simulink model "SCARA"  (R2018a)
settings: Solver=VariableStepAuto  StartTime=0.0  StopTime=10.0  RelTol=1e-3
model workspace: external: MATLAB File C:\Users\1511 MXTI\Desktop\CEFET\ROBÓTICA\SCARA 4\SCARA4_DataFile1.m (data not in the file)
undefined symbols (not defined in the file or in its folder): smiData, X, Y, Z
libraries: sm_lib x20, nesl_utility x9
(part 1 of 2)
settings Model: Creator=1511 MXTI  LastModifiedBy=1511 MXTI

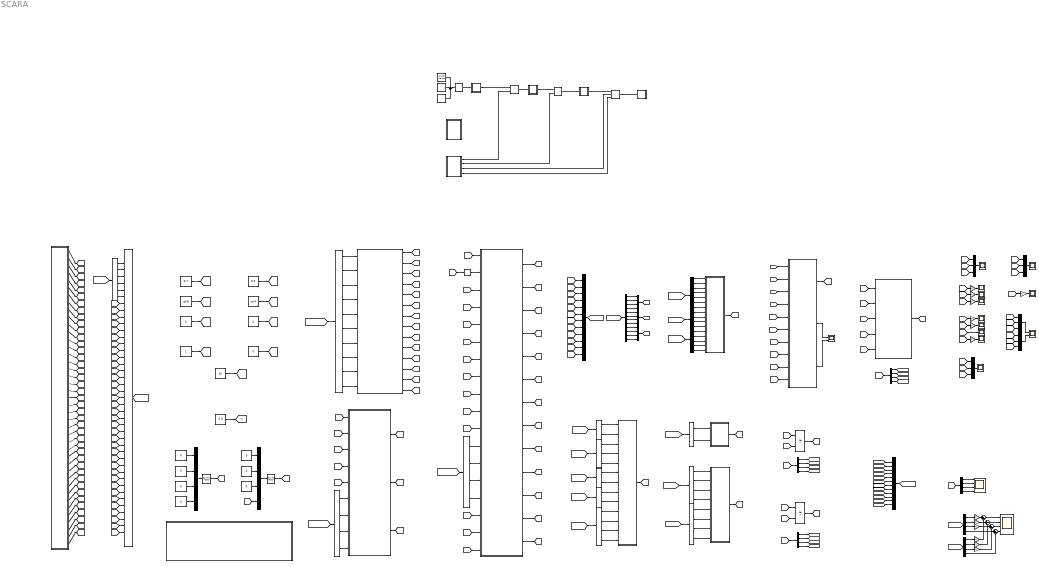
== system SCARA ==
  note: Disciplina: Robótica (GELE0931) 2020_2 T.A
      |
      | Professor: Luciano Raptopoulos
      | luciano.raptopoulos@cefet-rj.br
      |
      | Alunos:
      | Felipe Leite da Fonseca
      | Luan Almeida de Oliveira
      |
      | felipe.leite@aluno.cefet-rj.br
      |
      | luan.almeida@aluno.cefet-rj.br
  note: VELOCIDADES INICIAIS DAS JUNTAS
  note: TORQUE NAS JUNTAS
  note: DADOS DO MODELO
  note: TEST POSIÇÃO DA FERRAMENTA
  note: ANGULO DA FERRAMENTA
  note: Qs DESEJADOS
  note: POSIÇAO DA FERRAMENTA
  note: ACELERAÇÕES DA FERRAMENTA
  note: VELOCIDADES DA FERRAMENTA
  note: ANGULO DA FERRAMENTA
  note: DADOS DE ENTRADA DA TAREFA
  note: POSIÇÕES INICIAIS DAS JUNTAS
  note: VELOCIDADES SIMULADAS DAS JUNTAS
  note: POSIÇÕES SIMULADAS DAS JUNTAS
  note: CÁLCULO DA TRAJETÓRIA
  note: CINEMÁTICA INVERSA
  note: q dq ddq DESEJADOS
  note: q dq ddq SIMULADOS
  note: MODELO 3D DO SCARA
  note: SCARA COMPLETO
  note: TEMPO DE ASSENTAMENTO
  note: ERRO DAS JUNTAS
  note: PLOTAGENS
  note: PARAMETROS INICIAIS
  note: PARAMETROS FINAIS
  note: ALTURA DA FERRAMENTA EM RELAÇÃO AO SOLO
  note: DESEJADO
  note: SIMULADO
  note: INSTRUÇÕES DE UTILIZAÇÃO:
      |
      | Todos os grandes blocos utilizados para projetar o controle do robô SCARA apresentado foram separados nas áreas abaixo devidamente intituladas.
      |
      | As entradas estão dispostas na área em AZUL nos blocos de constante em VERDE .
      |
      | As saídas préviamente requisitadas serão abertas automáticamente ao rodar a simulação, como os torques, força e erros das juntas.
      |
      | Outras plotagens previamente definidas se encontram na área em AMARELO .
  note: M
  note: CONTROLADOR
  note: TESTE DA CINEMÁTICA
  note: TRATAMENTO DAS ENTRADAS
  note: DADOS DE ENTRADA DO CONTROLADOR
  note: PLANTA
  note: INTEGRAÇÕES
  note: G & D
  note: H
  Alpha final (rad) : Constant  Value=0
  Alpha inicial (rad) : Constant  Value=0
  Altura final (m) : Constant  Value=0
  Altura inicial (m) : Constant
  BASE_SCARA_2_RIGID : Subsystem
  Bus Creator : BusCreator  Inputs=12
  Bus Creator4 : BusCreator  Inputs=12
  Bus Creator5 : BusCreator  Inputs=41
  Bus Creator6 : BusCreator  Inputs=4
  Bus Creator7 : BusCreator  Inputs=4
  Bus Selector : BusSelector  OutputSignals=t,tf,R0,Rf,teta0,tetaf,alfa0,alfaf,h0,hf
  Bus Selector1 : BusSelector  OutputSignals=q1,q2,q4,q3
  Bus Selector10 : BusSelector  OutputSignals=L0,L1,e1,L2,e2,L3
  Bus Selector11 : BusSelector  OutputSignals=xG1,xG2,xG3,yG1,yG2,yG3
  Bus Selector12 : BusSelector  OutputSignals=signal2,signal4
  Bus Selector13 : BusSelector  OutputSignals=L1,L2
  Bus Selector14 : BusSelector  OutputSignals=signal1,signal2,signal4
  Bus Selector15 : BusSelector  OutputSignals=m2,m3
  Bus Selector16 : BusSelector  OutputSignals=xG2,xG3,yG2,yG3
  Bus Selector17 : BusSelector  OutputSignals=g,m3
  Bus Selector18 : BusSelector  OutputSignals=c1,c2,c3,c4
  Bus Selector19 : BusSelector  OutputSignals=signal2,signal4
  Bus Selector2 : BusSelector  OutputSignals=L0,L1,L2,e1
  Bus Selector20 : BusSelector  OutputSignals=signal5,signal6,signal7,signal8
  Bus Selector21 : BusSelector  OutputSignals=q1,q2,q3,q4,dq1d,dq2d,dq3d,dq4d,d2q1d,d2q2d,d2q3d,d2q4d
  Bus Selector3 : BusSelector  OutputSignals=signal1,signal2,signal4,signal3
  Bus Selector5 : BusSelector  OutputSignals=L0,L1,e1,L2
  Bus Selector9 : BusSelector  OutputSignals=Izz1,Izz2,Izz3,L1,L2,m1,m2,m3
  Bus to Vector1 : BusToVector
  Bus to Vector2 : BusToVector
  Cylindrical : sm_lib/Joints/Cylindrical Joint  SenseConstraintForce=off  SenseConstraintForceX=off  SenseConstraintForceY=off  SenseConstraintForceZ=off  SenseConstraintTorque=off  SenseConstraintTorqueX=off  SenseConstraintTorqueY=off  SenseConstraintTorqueZ=off  SenseTotalForce=off  SenseTotalForceX=off  SenseTotalForceY=off  SenseTotalForceZ=off  SenseTotalTorque=off  SenseTotalTorqueX=off  SenseTotalTorqueY=off  SenseTotalTorqueZ=off  CompositeWrenchDir=FollowerOnBase  CompositeWrenchFrame=BaseFrame  PzEquilibriumPosition=0  PzEquilibriumPositionUnits=m  PzSpringStiffness=0  PzSpringStiffnessUnits=N/m  PzDampingCoefficient=0  PzDampingCoefficientUnits=N/(m/s)  PzTorqueActuationMode=ComputedTorque  PzMotionActuationMode=InputMotion  PzSensePosition=off  PzSenseVelocity=off  PzSenseAcceleration=off  PzSenseTorqueForce=off  PzPositionTargetSpecify=on  PzPositionTargetPriority=Low  PzPositionTargetValue=smiData.CylindricalJoint(1).Pz.Pos  PzPositionTargetValueUnits=mm  PzVelocityTargetSpecify=off  PzVelocityTargetPriority=High  PzVelocityTargetValue=0  PzVelocityTargetValueUnits=m/s  RzEquilibriumPosition=0  RzEquilibriumPositionUnits=rad  RzSpringStiffness=0  RzSpringStiffnessUnits=N*m/rad  RzDampingCoefficient=0  RzDampingCoefficientUnits=N*m/(rad/s)  RzTorqueActuationMode=ComputedTorque  RzMotionActuationMode=InputMotion  RzSensePosition=off  RzSenseVelocity=off  RzSenseAcceleration=off  RzSenseTorqueForce=off  RzPositionTargetSpecify=on  RzPositionTargetPriority=Low  RzPositionTargetValue=smiData.CylindricalJoint(1).Rz.Pos  RzPositionTargetValueUnits=deg  RzVelocityTargetSpecify=off  RzVelocityTargetPriority=High  RzVelocityTargetValue=0  RzVelocityTargetValueUnits=deg/s
  D : MATLAB Function  TreatAsAtomicUnit=on
  DQ1S0 : Constant  Value=0
  DQ2S0 : Constant  Value=0
  DQ3S0 : Constant  Value=0
  DQ4S0 : Constant  Value=0
  Demux{,3..5} (4 alike) : Demux
  Duração da tarefa (s) : Constant  Value=10
  ELO_01_SCARA_1_RIGID : Subsystem
  ELO_02_SCARA_1_RIGID : Subsystem
  ELO_03_SCARA_1_RIGID : Subsystem
  G : MATLAB Function  TreatAsAtomicUnit=on
  Gain{,1..10,14..15} (13 alike) : Gain  Gain=180/pi
  H : MATLAB Function  TreatAsAtomicUnit=on
  Integrator2 : Integrator  InitialConditionSource=external  InitialCondition=[0 0 0 0]
  Integrator3 : Integrator  InitialConditionSource=external  InitialCondition=[0 0 0 0]
  JUNTAS DESEJADAS : Subsystem
  JUNTAS SIMULADAS : Subsystem
  M : MATLAB Function  TreatAsAtomicUnit=on
  MATLAB Function1 : MATLAB Function  TreatAsAtomicUnit=on
  MATLAB Function4 : MATLAB Function  TreatAsAtomicUnit=on
  MATLAB Function5 : MATLAB Function  TreatAsAtomicUnit=on
  MATLAB Function6 : MATLAB Function  TreatAsAtomicUnit=on
  MATLAB Function7 : MATLAB Function  TreatAsAtomicUnit=on
  MechanismConfiguration : sm_lib/Utilities/Mechanism Configuration  UniformGravity=Constant  GravityVector=[0 -9.80665 0]  GravityUnits=m/s^2  LinearizationDelta=0.001
  Memory : Memory
  Mux{,1..2,4..5} (5 alike) : Mux  Inputs=3
  Mux3 : Mux
  Mux7 : Mux
  Mux8 : Mux
  Q1S0 : Constant  Value=0
  Q2S0 : Constant  Value=0
  Q3S0 : Constant  Value=0
  Raio final (m) : Constant  Value=0.5
  Raio inicial (m) : Constant  Value=0.7
  Revolute : sm_lib/Joints/Revolute Joint  SenseConstraintForce=off  SenseConstraintForceX=off  SenseConstraintForceY=off  SenseConstraintForceZ=off  SenseConstraintTorque=off  SenseConstraintTorqueX=off  SenseConstraintTorqueY=off  SenseConstraintTorqueZ=off  SenseTotalForce=off  SenseTotalForceX=off  SenseTotalForceY=off  SenseTotalForceZ=off  SenseTotalTorque=off  SenseTotalTorqueX=off  SenseTotalTorqueY=off  SenseTotalTorqueZ=off  CompositeWrenchDir=FollowerOnBase  CompositeWrenchFrame=BaseFrame  EquilibriumPosition=0  EquilibriumPositionUnits=rad  SpringStiffness=0  SpringStiffnessUnits=N*m/rad  DampingCoefficient=0  DampingCoefficientUnits=N*m/(rad/s)  TorqueActuationMode=ComputedTorque  MotionActuationMode=InputMotion  SensePosition=off  SenseVelocity=off  SenseAcceleration=off  SenseTorqueForce=off  PositionTargetSpecify=on  PositionTargetPriority=Low  PositionTargetValue=smiData.RevoluteJoint(1).Rz.Pos  PositionTargetValueUnits=deg  VelocityTargetSpecify=off  VelocityTargetPriority=High  VelocityTargetValue=0  VelocityTargetValueUnits=deg/s
  Revolute1 : sm_lib/Joints/Revolute Joint  SenseConstraintForce=off  SenseConstraintForceX=off  SenseConstraintForceY=off  SenseConstraintForceZ=off  SenseConstraintTorque=off  SenseConstraintTorqueX=off  SenseConstraintTorqueY=off  SenseConstraintTorqueZ=off  SenseTotalForce=off  SenseTotalForceX=off  SenseTotalForceY=off  SenseTotalForceZ=off  SenseTotalTorque=off  SenseTotalTorqueX=off  SenseTotalTorqueY=off  SenseTotalTorqueZ=off  CompositeWrenchDir=FollowerOnBase  CompositeWrenchFrame=BaseFrame  EquilibriumPosition=0  EquilibriumPositionUnits=rad  SpringStiffness=0  SpringStiffnessUnits=N*m/rad  DampingCoefficient=0  DampingCoefficientUnits=N*m/(rad/s)  TorqueActuationMode=ComputedTorque  MotionActuationMode=InputMotion  SensePosition=off  SenseVelocity=off  SenseAcceleration=off  SenseTorqueForce=off  PositionTargetSpecify=on  PositionTargetPriority=Low  PositionTargetValue=smiData.RevoluteJoint(2).Rz.Pos  PositionTargetValueUnits=deg  VelocityTargetSpecify=off  VelocityTargetPriority=High  VelocityTargetValue=0  VelocityTargetValueUnits=deg/s
  Scope{,1..6,8..9,18..19} (11 alike) : Scope
  Scope10 : Scope  NumInputPorts=2
  Scope11 : Scope  NumInputPorts=4
  Scope15 : Scope  NumInputPorts=4
  Scope7 : Scope  NumInputPorts=2
  Solver Configuration : nesl_utility/Solver Configuration  PhysicalDomain=network_engine_domain  SubClassName=solver  LeftPortType=input  RightPortType=generic  Tones=[]  Harmonics=[]  SimulateNoise=off  Profile=off  UseLocalSampling=off  EnableSwitchedLinearOptims=on  FrequencyDomain=off  UseCCode=off  RelTol=0.001  AbsTol=1e-06  MinStep=1e-09  ToWorkspace=off  RevertToSquareIcSolve=off  NumHomotopyIterations=100  PhasorMode=off  PhasorModeNumHarmonics=1  DoDC=off  ResidualTolerance=1e-09  UseLocalSolver=off  LocalSolverChoice=NE_BACKWARD_EULER_ADVANCER  LocalSolverSampleTime=0.001  DoFixedCost=off  MaxNonlinIter=3  MaxModeIter=2  LinearAlgebra=Sparse  EquationFormulation=NE_TIME_EF  DelaysMemoryBudget=1024  AutomaticFiltering=on  FilteringTimeConstant=0.001
  Sum{,1..3} (4 alike) : Sum  Inputs=|+-
  TEMPO DE ASSENTAMENTO(s) : Constant  Value=0.5
  TRAMENTO DAS ENTRADAS : Subsystem
  Theta final (rad) : Constant  Value=-pi/4  OutMin=[-2*pi]  OutMax=[2*pi]
  Theta inicial (rad) : Constant  Value=-pi/8  OutMin=[-2*pi]  OutMax=[2*pi]
  Transform : sm_lib/Frames and Transforms/Rigid Transform  TranslationMethod=Cartesian  TranslationStandardOffset=0  TranslationLengthUnit=mm  TranslationStandardAxis=+Z  TranslationCartesianOffset=smiData.RigidTransform(7).translation  TranslationROffset=0  TranslationROffsetUnits=m  TranslationZOffset=0  TranslationZOffsetUnits=m  TranslationThetaOffset=0  TranslationThetaOffsetUnits=deg  RotationMethod=ArbitraryAxis  RotationAngleUnits=rad  RotationStandardAxis=+Z  RotationAngle=smiData.RigidTransform(7).angle  RotationArbitraryAxis=smiData.RigidTransform(7).axis  FollAlignAxisA=+X  BaseAlignAxisA=+Y  FollAlignAxisB=+Y  BaseAlignAxisB=+Z  RotationSequenceAxes=FollowerAxes  RotationSequence=XYX  RotationSequenceAngles=[0 0 0]  RotationSequenceAnglesUnits=deg  RotationMatrix=[1 0 0; 0 1 0; 0 0 1]
  VALORES : MATLAB Function  TreatAsAtomicUnit=on
  World : sm_lib/Frames and Transforms/World Frame
  tag scope: ALPHA_FINAL=global, ALPHA_INICIAL=global, ALTURA_FINAL=global, ALTURA_INICIAL=global, DURACAO_DA_TAREFA=global, L1i=global, L2i=global, L3i=global, LOi=global, P0s=global, RAIO_FINAL=global, RAIO_INICIAL=global, THETA_FINAL=global, THETA_INICIAL=global, Ts=global, V0s=global, c1=global, d2q1d=global, d2q2d=global, d2q3d=global, d2q4d=global, d2qs=global, ddy=global, dq1d=global, dq2d=global, dq3d=global, dq4d=global, dqs=global, e1i=global, e2i=global, horario=global, q1d=global, q2d=global, q3d=global, q4d=global, qd_dqd_d2qd=global, qs=global, qs_dqs_d2qs=global, t_x=global, t_y=global, t_z=global, teta=global, x=global, y=global, z=global
  wires:
  Bus Selector/5 -> MATLAB Function6/5(teta0)  "<teta0>"
  Bus Selector/8 -> MATLAB Function6/8(alfaf)  "<alfaf>"
  [INPUT] -> Bus Selector/1
  [x] -> MATLAB Function7/3(x)
  Bus Selector/1 -> MATLAB Function6/1(t)  "<t>"
  Bus Selector/6 -> MATLAB Function6/6(tetaf)  "<tetaf>"
  Bus Selector/3 -> MATLAB Function6/3(R0)  "<R0>"
  MATLAB Function6/5(z) -> [z]
  MATLAB Function6/13(dalfa) -> [dalfa]
  MATLAB Function6/1(horario) -> [horario]
  Bus Selector/2 -> MATLAB Function6/2(tf)  "<tf>"
  Bus Selector/4 -> MATLAB Function6/4(Rf)  "<Rf>"
  Bus Selector/7 -> MATLAB Function6/7(alfa0)  "<alfa0>"
  MATLAB Function6/11(ddz) -> [ddz]
  MATLAB Function6/6(dx) -> [dx]
  Bus Selector2/4 -> MATLAB Function7/15(e1)  "<e1>"
  MATLAB Function6/3(x) -> [x]
  MATLAB Function6/7(dy) -> [dy]
  MATLAB Function6/4(y) -> [y]
  MATLAB Function6/8(dz) -> [dz]
  [y] -> MATLAB Function7/4(y)
  MATLAB Function6/14(d2alfa) -> [ddalfa]
  Bus Selector2/2 -> MATLAB Function7/13(L1)  "<L1>"
  [alfa] -> MATLAB Function7/16(alfa)
  MATLAB Function6/2(teta) -> [teta]
  MATLAB Function6/9(ddx) -> [ddx]
  Bus Selector2/3 -> MATLAB Function7/14(L2)  "<L2>"
  [z] -> MATLAB Function7/5(z)
  MATLAB Function6/10(ddy) -> [ddy]
  MATLAB Function6/12(alfa) -> [alfa]
  Bus Selector2/1 -> MATLAB Function7/12(L0)  "<L0>"
  Memory/1 -> MATLAB Function7/2(phiAnterior)
  [phi] -> Memory/1
  [t_z] -> Mux5/3
  [t_x] -> Mux5/1
  [q2d] -> Gain4/1
  [t_y] -> Mux5/2
  [q4d] -> Gain2/1
  [z] -> Mux2/3
  Gain15/1 -> Scope4/1
  [y] -> Mux2/2
  Gain/1 -> Scope9/1
  Gain14/1 -> Scope3/1
  Gain1/1 -> Scope18/1
  Mux/1 -> Scope/1
  [ddz] -> Mux4/3
  Mux4/1 -> Scope2/1
  Gain2/1 -> Scope6/1
  [ddy] -> Mux4/2
  [ddx] -> Mux4/1
  [y] -> Mux/2
  Gain3/1 -> Scope19/1
  [x] -> Mux/1
  [dalfa] -> Gain1/1
  [dz] -> Mux1/3
  [dy] -> Mux1/2
  [q1d] -> Gain15/1
  Mux2/1 -> Scope7/1
  [dx] -> Mux1/1
  Mux1/1 -> Scope1/1
  [alfa] -> Gain/1
  Mux5/1 -> Scope7/2
  [z] -> Mux/3
  [x] -> Mux2/1
  [teta] -> Gain14/1
  [ddalfa] -> Gain3/1
  [q3d] -> Scope5/1
  Gain4/1 -> Scope8/1
  [q4d] -> MATLAB Function1/5(q4)
  Bus Selector5/1 -> MATLAB Function1/6(L0)  "<L0>"
  Bus Selector5/3 -> MATLAB Function1/8(e1)  "<e1>"
  [q3d] -> MATLAB Function1/4(q3)
  [q2d] -> MATLAB Function1/3(q2)
  Bus Selector5/2 -> MATLAB Function1/7(L1)  "<L1>"
  [DIMENSIONAL] -> Bus Selector5/1
  [horario] -> MATLAB Function1/1(horario)
  MATLAB Function1/1(x) -> [t_x]
  [q1d] -> MATLAB Function1/2(q1)
  MATLAB Function1/3(z) -> [t_z]
  Bus Selector5/4 -> MATLAB Function1/9(L2)  "<L2>"
  MATLAB Function1/2(y) -> [t_y]
  [q1d] -> Bus Creator4/1
  [q2d] -> Bus Creator4/2
  [q3d] -> Bus Creator4/3
  [q4d] -> Bus Creator4/4
  [dq1d] -> Bus Creator4/5
  [dq2d] -> Bus Creator4/6
  [dq3d] -> Bus Creator4/7
  [dq4d] -> Bus Creator4/8
  [d2q1d] -> Bus Creator4/9
  [d2q2d] -> Bus Creator4/10
  [d2q3d] -> Bus Creator4/11
  [d2q4d] -> Bus Creator4/12
  Bus Creator4/1 -> [qd_dqd_d2qd]
  Bus Selector14/2 -> H/4(dq2)  "<signal2>"
  Demux5/1 -> [d2q1s]
  Demux4/4 -> [q4s]
  Demux5/3 -> [d2q3s]
  [qs] -> MATLAB Function4/5(qs)
  Demux5/4 -> [d2q4s]
  Demux3/1 -> [dq1s]
  Demux5/2 -> [d2q2s]
  [dqs] -> MATLAB Function4/6(dqs)
  Demux3/3 -> [dq3s]
  Bus Selector14/1 -> H/3(dq1)  "<signal1>"
  Demux4/2 -> [q2s]
  Demux3/2 -> [dq2s]
  Demux4/3 -> [q3s]
  Demux4/1 -> [q1s]
  VALORES/2(L1i) -> [L1i]
  VALORES/3(e1i) -> [e1i]
  VALORES/4(L2i) -> [L2i]
  VALORES/5(e2i) -> [e2i]
  VALORES/6(L3i) -> [L3i]
  VALORES/7(c1) -> [c1]
  VALORES/8(c2) -> [c2]
  VALORES/9(c3) -> [c3]
  VALORES/10(c4) -> [c4]
  VALORES/11(g) -> [g]
  VALORES/12(m1) -> [m1]
  VALORES/13(xG1) -> [xG1]
  VALORES/14(yG1) -> [yG1]
  VALORES/15(zG1) -> [zG1]
  VALORES/16(Ixx1) -> [Ixx1]
  VALORES/17(Ixy1) -> [Ixy1]
  VALORES/18(Ixz1) -> [Ixz1]
  VALORES/19(Iyy1) -> [Iyy1]
  VALORES/20(Iyz1) -> [Iyz1]
  VALORES/21(Izz1) -> [Izz1]
  VALORES/22(m2) -> [m2]
  VALORES/23(xG2) -> [xG2]
  VALORES/24(yG2) -> [yG2]
  VALORES/25(zG2) -> [zG2]
  VALORES/26(Ixx2) -> [Ixx2]
  VALORES/27(Ixy2) -> [Ixy2]
  VALORES/28(Ixz2) -> [Ixz2]
  VALORES/29(Iyy2) -> [Iyy2]
  VALORES/30(Iyz2) -> [Iyz2]
  VALORES/31(Izz2) -> [Izz2]
  VALORES/32(m3) -> [m3]
  VALORES/41(Izz3) -> [Izz3]
  VALORES/40(Iyz3) -> [Iyz3]
  VALORES/39(Iyy3) -> [Iyy3]
  VALORES/38(Ixz3) -> [Ixz3]
  VALORES/37(Ixy3) -> [Ixy3]
  VALORES/36(Ixx3) -> [Ixx3]
  VALORES/35(zG3) -> [zG3]
  VALORES/34(yG3) -> [yG3]
  VALORES/33(xG3) -> [xG3]
  VALORES/1(LOi) -> [LOi]
  [c1] -> Bus Creator5/7
  [c2] -> Bus Creator5/8
  [c3] -> Bus Creator5/9
  [c4] -> Bus Creator5/10
  [g] -> Bus Creator5/11
  [m1] -> Bus Creator5/12
  [xG1] -> Bus Creator5/13
  [Ixz1] -> Bus Creator5/18
  [Ixy1] -> Bus Creator5/17
  [Ixx1] -> Bus Creator5/16
  [zG1] -> Bus Creator5/15
  [yG1] -> Bus Creator5/14
  [Iyy1] -> Bus Creator5/19
  [Iyz1] -> Bus Creator5/20
  [Izz1] -> Bus Creator5/21
  [m2] -> Bus Creator5/22
  [xG2] -> Bus Creator5/23
  [yG2] -> Bus Creator5/24
  [Ixx2] -> Bus Creator5/26
  [zG2] -> Bus Creator5/25
  [Ixy2] -> Bus Creator5/27
  [Ixz2] -> Bus Creator5/28
  [Iyy2] -> Bus Creator5/29
  [Iyz2] -> Bus Creator5/30
  [Izz2] -> Bus Creator5/31
  [m3] -> Bus Creator5/32
  [xG3] -> Bus Creator5/33
  [yG3] -> Bus Creator5/34
  [zG3] -> Bus Creator5/35
  [Ixx3] -> Bus Creator5/36
  [Ixy3] -> Bus Creator5/37
  [Ixz3] -> Bus Creator5/38
  [Iyy3] -> Bus Creator5/39
  [Iyz3] -> Bus Creator5/40
  [Izz3] -> Bus Creator5/41
  Bus Creator5/1 -> [ALL_IN]
  [ALL_IN] -> Bus Selector9/1
  [DIMENSIONAL] -> Bus Selector10/1
  Bus Selector10/1 -> Bus Creator5/1  "<L0>"
  Bus Selector10/2 -> Bus Creator5/2  "<L1>"
  Bus Selector10/3 -> Bus Creator5/3  "<e1>"
  Bus Selector10/4 -> Bus Creator5/4  "<L2>"
  Bus Selector10/5 -> Bus Creator5/5  "<e2>"
  Bus Selector10/6 -> Bus Creator5/6  "<L3>"
  Bus Selector9/1 -> M/1(Izz1)  "<Izz1>"
  Bus Selector9/2 -> M/2(Izz2)  "<Izz2>"
  Bus Selector9/3 -> M/3(Izz3)  "<Izz3>"
  Bus Selector9/4 -> M/4(L1)  "<L1>"
  Bus Selector9/5 -> M/5(L2)  "<L2>"
  Bus Selector9/6 -> M/6(m1)  "<m1>"
  Bus Selector9/7 -> M/7(m2)  "<m2>"
  Bus Selector9/8 -> M/8(m3)  "<m3>"
  [ALL_IN] -> Bus Selector11/1
  Bus Selector11/1 -> M/11(xG1)  "<xG1>"
  Bus Selector11/2 -> M/12(xG2)  "<xG2>"
  Bus Selector11/3 -> M/13(xG3)  "<xG3>"
  Bus Selector11/4 -> M/14(yG1)  "<yG1>"
  Bus Selector11/5 -> M/15(yG2)  "<yG2>"
  Bus Selector11/6 -> M/16(yG3)  "<yG3>"
  [dq2s] -> Bus Creator/6
  [dq1s] -> Bus Creator/5
  [dq3s] -> Bus Creator/7
  [dq4s] -> Bus Creator/8
  [d2q2s] -> Bus Creator/10
  [d2q3s] -> Bus Creator/11
  [d2q4s] -> Bus Creator/12
  [d2q1s] -> Bus Creator/9
  Bus Creator/1 -> [qs_dqs_d2qs]
  [q1s] -> Bus Creator/1
  [q2s] -> Bus Creator/2
  [q3s] -> Bus Creator/3
  [q4s] -> Bus Creator/4
  Demux3/4 -> [dq4s]
  [qs_dqs_d2qs] -> Bus Selector12/1
  Bus Selector12/1 -> M/9(q2)  "<signal2>"
  Bus Selector12/2 -> M/10(q4)  "<signal4>"
  [M] -> MATLAB Function5/1(M)
  [M] -> MATLAB Function4/7(M)
  M/1(M) -> [M]
  [ALL_IN] -> Bus Selector13/1
  Bus Selector13/1 -> H/1(L1)  "<L1>"
  Bus Selector13/2 -> H/2(L2)  "<L2>"
  [qs_dqs_d2qs] -> Bus Selector14/1
  Bus Selector14/3 -> H/5(dq4)  "<signal4>"
  [ALL_IN] -> Bus Selector15/1
  Bus Selector15/1 -> H/6(m2)  "<m2>"
  Bus Selector15/2 -> H/7(m3)  "<m3>"
  [ALL_IN] -> Bus Selector16/1
  Bus Selector16/1 -> H/10(xG2)  "<xG2>"
  Bus Selector16/2 -> H/11(xG3)  "<xG3>"
  Bus Selector16/3 -> H/12(yG2)  "<yG2>"
  Bus Selector16/4 -> H/13(yG3)  "<yG3>"
  [ALL_IN] -> Bus Selector17/1
  Bus Selector17/1 -> G/1(g)  "<g>"
  Bus Selector17/2 -> G/2(m3)  "<m3>"
  [ALL_IN] -> Bus Selector18/1
  Bus Selector18/1 -> D/1(c1)  "<c1>"
  Bus Selector18/2 -> D/2(c2)  "<c2>"
  Bus Selector18/3 -> D/3(c3)  "<c3>"
  Bus Selector18/4 -> D/4(c4)  "<c4>"
  [qs_dqs_d2qs] -> Bus Selector19/1
  Bus Selector19/1 -> H/8(q2)  "<signal2>"
  Bus Selector19/2 -> H/9(q4)  "<signal4>"
  [qs_dqs_d2qs] -> Bus Selector20/1
  Bus Selector20/1 -> D/5(dq1)  "<signal5>"
  Bus Selector20/2 -> D/6(dq2)  "<signal6>"
  Bus Selector20/3 -> D/7(dq3)  "<signal7>"
  Bus Selector20/4 -> D/8(dq4)  "<signal8>"
  H/1(H) -> [H]
  [H] -> MATLAB Function4/8(H)
  [H] -> MATLAB Function5/3(H)
  G/1(G) -> [G]
  [G] -> MATLAB Function4/9(G)
  [G] -> MATLAB Function5/4(G)
  D/1(D) -> [D]
  [D] -> MATLAB Function4/10(D)
  [D] -> MATLAB Function5/5(D)
  MATLAB Function4/1(Tc) -> [Tc]
  [Tc] -> MATLAB Function5/2(Tc)
  Bus Selector21/1 -> Mux3/1  "<q1>"
  Bus Selector21/2 -> Mux3/2  "<q2>"
  Bus Selector21/3 -> Mux3/3  "<q3>"
  Bus Selector21/4 -> Mux3/4  "<q4>"
  [qd_dqd_d2qd] -> Bus Selector21/1
  Bus Selector21/5 -> Mux7/1  "<dq1d>"
  Bus Selector21/6 -> Mux7/2  "<dq2d>"
  Bus Selector21/7 -> Mux7/3  "<dq3d>"
  Bus Selector21/8 -> Mux7/4  "<dq4d>"
  Bus Selector21/9 -> Mux8/1  "<d2q1d>"
  Bus Selector21/10 -> Mux8/2  "<d2q2d>"
  Bus Selector21/11 -> Mux8/3  "<d2q3d>"
  Bus Selector21/12 -> Mux8/4  "<d2q4d>"
  Mux3/1 -> [qd]
  Mux7/1 -> [dqd]
  Mux8/1 -> [d2qd]
  [d2qd] -> MATLAB Function4/4(d2qd)
  [dqd] -> MATLAB Function4/3(dqd)
  [qd] -> MATLAB Function4/2(qd)
  MATLAB Function5/1(d2qs) -> [d2qs]
  Bus Creator6/1 -> Bus to Vector1/1
  Bus to Vector1/1 -> [V0s]
  DQ1S0/1 -> Bus Creator6/1
  Bus Creator7/1 -> Bus to Vector2/1
  Q3S0/1 -> Bus Creator7/3
  [alfa0] -> Bus Creator7/4
  Q1S0/1 -> Bus Creator7/1
  Q2S0/1 -> Bus Creator7/2
  Bus to Vector2/1 -> [P0s]
  [V0s] -> Integrator3/2
  [d2qs] -> Integrator3/1
  Integrator3/1 -> [dqs]
  [dqs] -> Integrator2/1
  [P0s] -> Integrator2/2
  Integrator2/1 -> [qs]
  [d2qs] -> Demux5/1
  [dqs] -> Demux3/1
  [qs] -> Demux4/1
  Bus Selector/9 -> MATLAB Function6/9(h0)  "<h0>"
  Bus Selector/10 -> MATLAB Function6/10(hf)  "<hf>"
  MATLAB Function7/6(dq1d) -> [dq1d]
  MATLAB Function7/7(dq2d) -> [dq2d]
  MATLAB Function7/8(dq3d) -> [dq3d]
  MATLAB Function7/9(dq4d) -> [dq4d]
  MATLAB Function7/1(phi) -> [phi]
  MATLAB Function7/2(q1) -> [q1d]
  MATLAB Function7/3(q2) -> [q2d]
  MATLAB Function7/4(q3) -> [q3d]
  MATLAB Function7/5(q4) -> [q4d]
  [horario] -> MATLAB Function7/1(horario)
  [DIMENSIONAL] -> Bus Selector2/1
  [dalfa] -> MATLAB Function7/17(dalfa)
  [ddalfa] -> MATLAB Function7/18(ddalfa)
  MATLAB Function7/10(d2q1d) -> [d2q1d]
  MATLAB Function7/11(d2q2d) -> [d2q2d]
  MATLAB Function7/12(d2q3d) -> [d2q3d]
  MATLAB Function7/13(d2q4d) -> [d2q4d]
  [dx] -> MATLAB Function7/6(dx)
  [dy] -> MATLAB Function7/7(dy)
  [dz] -> MATLAB Function7/8(dz)
  [ddx] -> MATLAB Function7/9(d2x)
  [ddy] -> MATLAB Function7/10(d2y)
  [ddz] -> MATLAB Function7/11(d2z)
  [Ts] -> MATLAB Function4/1(Ts)
  TEMPO DE ASSENTAMENTO(s)/1 -> [Ts]
  Sum/1 -> Scope11/1
  MATLAB Function4/2(Kp) -> Scope10/1
  MATLAB Function4/3(Kd) -> Scope10/2
  [qd_dqd_d2qd] -> Bus Selector1/1
  Bus Selector1/1 -> Gain5/1  "<q1>"
  Bus Selector1/2 -> Gain7/1  "<q2>"
  Bus Selector1/3 -> Gain8/1  "<q4>"
  Gain5/1 -> Sum/1
  Bus Selector3/3 -> Gain10/1  "<signal4>"
  Bus Selector3/2 -> Gain9/1  "<signal2>"
  Bus Selector3/1 -> Gain6/1  "<signal1>"
  [qs_dqs_d2qs] -> Bus Selector3/1
  Gain6/1 -> Sum/2
  Gain7/1 -> Sum1/1
  Gain9/1 -> Sum1/2
  Sum1/1 -> Scope11/2
  Gain8/1 -> Sum2/1
  Gain10/1 -> Sum2/2
  Sum2/1 -> Scope11/3
  Bus Selector3/4 -> Sum3/2  "<signal3>"
  Bus Selector1/4 -> Sum3/1  "<q3>"
  Sum3/1 -> Scope11/4
  [Tc] -> Demux/1
  Demux/1 -> Scope15/1
  Demux/2 -> Scope15/2
  Demux/3 -> Scope15/3
  Demux/4 -> Scope15/4
  Raio inicial (m)/1 -> [RAIO_INICIAL]
  Theta inicial (rad)/1 -> [THETA_INICIAL]
  Alpha inicial (rad)/1 -> [ALPHA_INICIAL]
  Altura inicial (m)/1 -> [ALTURA_INICIAL]
  Altura final (m)/1 -> [ALTURA_FINAL]
  Alpha final (rad)/1 -> [ALPHA_FINAL]
  Theta final (rad)/1 -> [THETA_FINAL]
  Raio final (m)/1 -> [RAIO_FINAL]
  Duração da tarefa (s)/1 -> [DURACAO_DA_TAREFA]
  DQ2S0/1 -> Bus Creator6/2
  DQ3S0/1 -> Bus Creator6/3
  DQ4S0/1 -> Bus Creator6/4
  connections:
  Transform/LConn1 -- MechanismConfiguration/RConn1 -- Solver Configuration/RConn1 -- World/RConn1
  ELO_01_SCARA_1_RIGID/RConn1 -- Revolute/LConn1
  ELO_02_SCARA_1_RIGID/LConn1 -- Revolute/RConn1
  Cylindrical/LConn1 -- ELO_02_SCARA_1_RIGID/RConn1
  Cylindrical/RConn1 -- ELO_03_SCARA_1_RIGID/LConn1
  BASE_SCARA_2_RIGID/RConn1 -- Revolute1/LConn1
  ELO_01_SCARA_1_RIGID/LConn1 -- Revolute1/RConn1
  BASE_SCARA_2_RIGID/LConn1 -- Transform/RConn1
  JUNTAS SIMULADAS/RConn2 -- Revolute/LConn2
  JUNTAS SIMULADAS/RConn3 -- Cylindrical/LConn2
  JUNTAS SIMULADAS/RConn4 -- Cylindrical/LConn3
  JUNTAS SIMULADAS/RConn1 -- Revolute1/LConn2

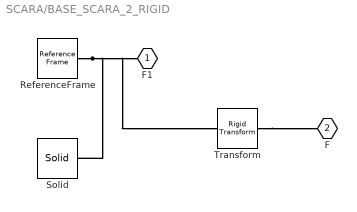
== system SCARA/BASE_SCARA_2_RIGID ==
  ReferenceFrame : sm_lib/Frames and Transforms/Reference Frame
  Solid : sm_lib/Body Elements/Solid  InertiaType=Custom  Mass=smiData.Solid(2).mass  MassUnits=kg  CenterOfMass=smiData.Solid(2).CoM  CenterOfMassUnits=mm  MomentsOfInertia=smiData.Solid(2).MoI  MomentsOfInertiaUnits=kg*mm^2  ProductsOfInertia=smiData.Solid(2).PoI  ProductsOfInertiaUnits=kg*mm^2  DensityBased=on  Density=1000  DensityUnits=kg/m^3  DoExposeReferenceFrame=on  SerializedFrames=<Frames/>  GraphicType=FromGeometry  MarkerShape=Sphere  MarkerSize=10  GraphicVisPropType=SimpleVisualProperties  GraphicDiffuseColor=smiData.Solid(2).color  GraphicSpecularColor=[0.5 0.5 0.5 1.0]  GraphicAmbientColor=[0.15 0.15 0.15 1.0]  GraphicEmissiveColor=[0.0 0.0 0.0 1.0]  GraphicShininess=75  GraphicOpacity=smiData.Solid(2).opacity  GeometryShape=FromFile  RectangleSize=[1 1]  RectangleSizeUnits=m  BrickDimensions=[1 1 1]  BrickDimensionUnits=m  CylinderRadius=1  CylinderRadiusUnits=m  CylinderLength=1  CylinderLengthUnits=m  SphereRadius=1  SphereRadiusUnits=m  EllipsoidRadii=[1 1 1]  EllipsoidRadiiUnits=m  ExtrusionCrossSection=[1 1; -1 1; -1 -1; 1 -1]  ExtrusionCrossSectionUnits=m  ExtrusionLength=1  ExtrusionLengthUnits=m  PolygonNumSides=3  PolygonOuterRadius=1  PolygonOuterRadiusUnits=m  ExtGeomFileType=STEP  ExtGeomFileName=BASE SCARA_Valor predeterminado_sldprt.STEP  ExtGeomFileUnits=m  RevolutionCrossSection=[1 1; 1 -1; 2 -1; 2 1]  RevolutionCrossSectionUnits=m  RevolutionExtent=Full  RevolutionAngle=180  RevolutionAngleUnits=deg
  Transform : sm_lib/Frames and Transforms/Rigid Transform  TranslationMethod=Cartesian  TranslationStandardOffset=0  TranslationLengthUnit=mm  TranslationStandardAxis=+Z  TranslationCartesianOffset=smiData.RigidTransform(5).translation  TranslationROffset=0  TranslationROffsetUnits=m  TranslationZOffset=0  TranslationZOffsetUnits=m  TranslationThetaOffset=0  TranslationThetaOffsetUnits=deg  RotationMethod=ArbitraryAxis  RotationAngleUnits=rad  RotationStandardAxis=+Z  RotationAngle=smiData.RigidTransform(5).angle  RotationArbitraryAxis=smiData.RigidTransform(5).axis  FollAlignAxisA=+X  BaseAlignAxisA=+Y  FollAlignAxisB=+Y  BaseAlignAxisB=+Z  RotationSequenceAxes=FollowerAxes  RotationSequence=XYX  RotationSequenceAngles=[0 0 0]  RotationSequenceAnglesUnits=deg  RotationMatrix=[1 0 0; 0 1 0; 0 0 1]
  F1 : PMIOPort  Side=Left
  F : PMIOPort  Port=2  Side=Right
  connections:
  Solid/RConn1 -- ReferenceFrame/RConn1 -- Transform/LConn1 -- F1/RConn1
  Transform/RConn1 -- F/RConn1

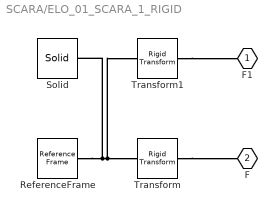
== system SCARA/ELO_01_SCARA_1_RIGID ==
  ReferenceFrame : sm_lib/Frames and Transforms/Reference Frame
  Solid : sm_lib/Body Elements/Solid  InertiaType=Custom  Mass=smiData.Solid(3).mass  MassUnits=kg  CenterOfMass=smiData.Solid(3).CoM  CenterOfMassUnits=mm  MomentsOfInertia=smiData.Solid(3).MoI  MomentsOfInertiaUnits=kg*mm^2  ProductsOfInertia=smiData.Solid(3).PoI  ProductsOfInertiaUnits=kg*mm^2  DensityBased=on  Density=1000  DensityUnits=kg/m^3  DoExposeReferenceFrame=on  SerializedFrames=<Frames/>  GraphicType=FromGeometry  MarkerShape=Sphere  MarkerSize=10  GraphicVisPropType=SimpleVisualProperties  GraphicDiffuseColor=smiData.Solid(3).color  GraphicSpecularColor=[0.5 0.5 0.5 1.0]  GraphicAmbientColor=[0.15 0.15 0.15 1.0]  GraphicEmissiveColor=[0.0 0.0 0.0 1.0]  GraphicShininess=75  GraphicOpacity=smiData.Solid(3).opacity  GeometryShape=FromFile  RectangleSize=[1 1]  RectangleSizeUnits=m  BrickDimensions=[1 1 1]  BrickDimensionUnits=m  CylinderRadius=1  CylinderRadiusUnits=m  CylinderLength=1  CylinderLengthUnits=m  SphereRadius=1  SphereRadiusUnits=m  EllipsoidRadii=[1 1 1]  EllipsoidRadiiUnits=m  ExtrusionCrossSection=[1 1; -1 1; -1 -1; 1 -1]  ExtrusionCrossSectionUnits=m  ExtrusionLength=1  ExtrusionLengthUnits=m  PolygonNumSides=3  PolygonOuterRadius=1  PolygonOuterRadiusUnits=m  ExtGeomFileType=STEP  ExtGeomFileName=ELO 01 SCARA_Valor predeterminado_sldprt.STEP  ExtGeomFileUnits=m  RevolutionCrossSection=[1 1; 1 -1; 2 -1; 2 1]  RevolutionCrossSectionUnits=m  RevolutionExtent=Full  RevolutionAngle=180  RevolutionAngleUnits=deg
  Transform : sm_lib/Frames and Transforms/Rigid Transform  TranslationMethod=Cartesian  TranslationStandardOffset=0  TranslationLengthUnit=mm  TranslationStandardAxis=+Z  TranslationCartesianOffset=smiData.RigidTransform(1).translation  TranslationROffset=0  TranslationROffsetUnits=m  TranslationZOffset=0  TranslationZOffsetUnits=m  TranslationThetaOffset=0  TranslationThetaOffsetUnits=deg  RotationMethod=AlignedAxes  RotationAngleUnits=rad  RotationStandardAxis=+Z  RotationAngle=smiData.RigidTransform(1).angle  RotationArbitraryAxis=smiData.RigidTransform(1).axis  FollAlignAxisA=+X  BaseAlignAxisA=+X  FollAlignAxisB=+Y  BaseAlignAxisB=+Y  RotationSequenceAxes=FollowerAxes  RotationSequence=XYX  RotationSequenceAngles=[0 0 0]  RotationSequenceAnglesUnits=deg  RotationMatrix=[1 0 0; 0 1 0; 0 0 1]
  Transform1 : sm_lib/Frames and Transforms/Rigid Transform  TranslationMethod=Cartesian  TranslationStandardOffset=0  TranslationLengthUnit=mm  TranslationStandardAxis=+Z  TranslationCartesianOffset=smiData.RigidTransform(6).translation  TranslationROffset=0  TranslationROffsetUnits=m  TranslationZOffset=0  TranslationZOffsetUnits=m  TranslationThetaOffset=0  TranslationThetaOffsetUnits=deg  RotationMethod=ArbitraryAxis  RotationAngleUnits=rad  RotationStandardAxis=+Z  RotationAngle=smiData.RigidTransform(6).angle  RotationArbitraryAxis=smiData.RigidTransform(6).axis  FollAlignAxisA=+X  BaseAlignAxisA=+Y  FollAlignAxisB=+Y  BaseAlignAxisB=+Z  RotationSequenceAxes=FollowerAxes  RotationSequence=XYX  RotationSequenceAngles=[0 0 0]  RotationSequenceAnglesUnits=deg  RotationMatrix=[1 0 0; 0 1 0; 0 0 1]
  F1 : PMIOPort  Side=Left
  F : PMIOPort  Port=2  Side=Right
  connections:
  Solid/RConn1 -- ReferenceFrame/RConn1 -- Transform/LConn1 -- Transform1/LConn1
  Transform/RConn1 -- F/RConn1
  Transform1/RConn1 -- F1/RConn1

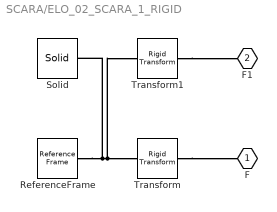
== system SCARA/ELO_02_SCARA_1_RIGID ==
  ReferenceFrame : sm_lib/Frames and Transforms/Reference Frame
  Solid : sm_lib/Body Elements/Solid  InertiaType=Custom  Mass=smiData.Solid(1).mass  MassUnits=kg  CenterOfMass=smiData.Solid(1).CoM  CenterOfMassUnits=mm  MomentsOfInertia=smiData.Solid(1).MoI  MomentsOfInertiaUnits=kg*mm^2  ProductsOfInertia=smiData.Solid(1).PoI  ProductsOfInertiaUnits=kg*mm^2  DensityBased=on  Density=1000  DensityUnits=kg/m^3  DoExposeReferenceFrame=on  SerializedFrames=<Frames/>  GraphicType=FromGeometry  MarkerShape=Sphere  MarkerSize=10  GraphicVisPropType=SimpleVisualProperties  GraphicDiffuseColor=smiData.Solid(1).color  GraphicSpecularColor=[0.5 0.5 0.5 1.0]  GraphicAmbientColor=[0.15 0.15 0.15 1.0]  GraphicEmissiveColor=[0.0 0.0 0.0 1.0]  GraphicShininess=75  GraphicOpacity=smiData.Solid(1).opacity  GeometryShape=FromFile  RectangleSize=[1 1]  RectangleSizeUnits=m  BrickDimensions=[1 1 1]  BrickDimensionUnits=m  CylinderRadius=1  CylinderRadiusUnits=m  CylinderLength=1  CylinderLengthUnits=m  SphereRadius=1  SphereRadiusUnits=m  EllipsoidRadii=[1 1 1]  EllipsoidRadiiUnits=m  ExtrusionCrossSection=[1 1; -1 1; -1 -1; 1 -1]  ExtrusionCrossSectionUnits=m  ExtrusionLength=1  ExtrusionLengthUnits=m  PolygonNumSides=3  PolygonOuterRadius=1  PolygonOuterRadiusUnits=m  ExtGeomFileType=STEP  ExtGeomFileName=ELO 02 SCARA_Valor predeterminado_sldprt.STEP  ExtGeomFileUnits=m  RevolutionCrossSection=[1 1; 1 -1; 2 -1; 2 1]  RevolutionCrossSectionUnits=m  RevolutionExtent=Full  RevolutionAngle=180  RevolutionAngleUnits=deg
  Transform : sm_lib/Frames and Transforms/Rigid Transform  TranslationMethod=Cartesian  TranslationStandardOffset=0  TranslationLengthUnit=mm  TranslationStandardAxis=+Z  TranslationCartesianOffset=smiData.RigidTransform(2).translation  TranslationROffset=0  TranslationROffsetUnits=m  TranslationZOffset=0  TranslationZOffsetUnits=m  TranslationThetaOffset=0  TranslationThetaOffsetUnits=deg  RotationMethod=AlignedAxes  RotationAngleUnits=rad  RotationStandardAxis=+Z  RotationAngle=smiData.RigidTransform(2).angle  RotationArbitraryAxis=smiData.RigidTransform(2).axis  FollAlignAxisA=+Z  BaseAlignAxisA=+Z  FollAlignAxisB=+Y  BaseAlignAxisB=+Y  RotationSequenceAxes=FollowerAxes  RotationSequence=XYX  RotationSequenceAngles=[0 0 0]  RotationSequenceAnglesUnits=deg  RotationMatrix=[1 0 0; 0 1 0; 0 0 1]
  Transform1 : sm_lib/Frames and Transforms/Rigid Transform  TranslationMethod=Cartesian  TranslationStandardOffset=0  TranslationLengthUnit=mm  TranslationStandardAxis=+Z  TranslationCartesianOffset=smiData.RigidTransform(3).translation  TranslationROffset=0  TranslationROffsetUnits=m  TranslationZOffset=0  TranslationZOffsetUnits=m  TranslationThetaOffset=0  TranslationThetaOffsetUnits=deg  RotationMethod=AlignedAxes  RotationAngleUnits=rad  RotationStandardAxis=+Z  RotationAngle=smiData.RigidTransform(3).angle  RotationArbitraryAxis=smiData.RigidTransform(3).axis  FollAlignAxisA=+Z  BaseAlignAxisA=+Z  FollAlignAxisB=+Y  BaseAlignAxisB=+Y  RotationSequenceAxes=FollowerAxes  RotationSequence=XYX  RotationSequenceAngles=[0 0 0]  RotationSequenceAnglesUnits=deg  RotationMatrix=[1 0 0; 0 1 0; 0 0 1]
  F : PMIOPort  Side=Left
  F1 : PMIOPort  Port=2  Side=Right
  connections:
  Solid/RConn1 -- ReferenceFrame/RConn1 -- Transform/LConn1 -- Transform1/LConn1
  Transform/RConn1 -- F/RConn1
  Transform1/RConn1 -- F1/RConn1

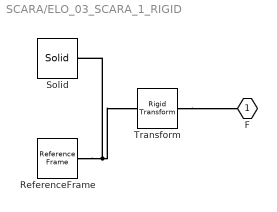
== system SCARA/ELO_03_SCARA_1_RIGID ==
  ReferenceFrame : sm_lib/Frames and Transforms/Reference Frame
  Solid : sm_lib/Body Elements/Solid  InertiaType=Custom  Mass=smiData.Solid(4).mass  MassUnits=kg  CenterOfMass=smiData.Solid(4).CoM  CenterOfMassUnits=mm  MomentsOfInertia=smiData.Solid(4).MoI  MomentsOfInertiaUnits=kg*mm^2  ProductsOfInertia=smiData.Solid(4).PoI  ProductsOfInertiaUnits=kg*mm^2  DensityBased=on  Density=1000  DensityUnits=kg/m^3  DoExposeReferenceFrame=on  SerializedFrames=<Frames/>  GraphicType=FromGeometry  MarkerShape=Sphere  MarkerSize=10  GraphicVisPropType=SimpleVisualProperties  GraphicDiffuseColor=smiData.Solid(4).color  GraphicSpecularColor=[0.5 0.5 0.5 1.0]  GraphicAmbientColor=[0.15 0.15 0.15 1.0]  GraphicEmissiveColor=[0.0 0.0 0.0 1.0]  GraphicShininess=75  GraphicOpacity=smiData.Solid(4).opacity  GeometryShape=FromFile  RectangleSize=[1 1]  RectangleSizeUnits=m  BrickDimensions=[1 1 1]  BrickDimensionUnits=m  CylinderRadius=1  CylinderRadiusUnits=m  CylinderLength=1  CylinderLengthUnits=m  SphereRadius=1  SphereRadiusUnits=m  EllipsoidRadii=[1 1 1]  EllipsoidRadiiUnits=m  ExtrusionCrossSection=[1 1; -1 1; -1 -1; 1 -1]  ExtrusionCrossSectionUnits=m  ExtrusionLength=1  ExtrusionLengthUnits=m  PolygonNumSides=3  PolygonOuterRadius=1  PolygonOuterRadiusUnits=m  ExtGeomFileType=STEP  ExtGeomFileName=ELO 03 SCARA_Valor predeterminado_sldprt.STEP  ExtGeomFileUnits=m  RevolutionCrossSection=[1 1; 1 -1; 2 -1; 2 1]  RevolutionCrossSectionUnits=m  RevolutionExtent=Full  RevolutionAngle=180  RevolutionAngleUnits=deg
  Transform : sm_lib/Frames and Transforms/Rigid Transform  TranslationMethod=Cartesian  TranslationStandardOffset=0  TranslationLengthUnit=mm  TranslationStandardAxis=+Z  TranslationCartesianOffset=smiData.RigidTransform(4).translation  TranslationROffset=0  TranslationROffsetUnits=m  TranslationZOffset=0  TranslationZOffsetUnits=m  TranslationThetaOffset=0  TranslationThetaOffsetUnits=deg  RotationMethod=AlignedAxes  RotationAngleUnits=rad  RotationStandardAxis=+Z  RotationAngle=smiData.RigidTransform(4).angle  RotationArbitraryAxis=smiData.RigidTransform(4).axis  FollAlignAxisA=+X  BaseAlignAxisA=+X  FollAlignAxisB=+Y  BaseAlignAxisB=+Y  RotationSequenceAxes=FollowerAxes  RotationSequence=XYX  RotationSequenceAngles=[0 0 0]  RotationSequenceAnglesUnits=deg  RotationMatrix=[1 0 0; 0 1 0; 0 0 1]
  F : PMIOPort  Side=Left
  connections:
  Solid/RConn1 -- ReferenceFrame/RConn1 -- Transform/LConn1
  Transform/RConn1 -- F/RConn1

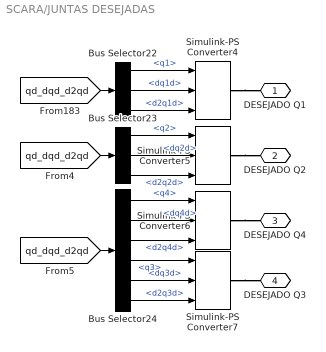
== system SCARA/JUNTAS DESEJADAS ==
  Bus Selector22 : BusSelector  OutputSignals=q1,dq1d,d2q1d
  Bus Selector23 : BusSelector  OutputSignals=q2,dq2d,d2q2d
  Bus Selector24 : BusSelector  OutputSignals=q4,dq4d,d2q4d,q3,dq3d,d2q3d
  Simulink-PS Converter{4..7} (4 alike) : nesl_utility/Simulink-PS Converter  PhysicalDomain=network_engine_domain  SubClassName=ps_input  LeftPortType=input  RightPortType=output  PseudoPeriodic=off  Frequencies=[]  NoiseDistribution=none  NoiseParameters=[]  Unit=1  AffineConversion=off  FilteringAndDerivatives=provide  SimscapeFilterOrder=1  InputFilterTimeConstant=0.001  UdotUserProvided=2
  DESEJADO Q1 : PMIOPort  Side=Right
  DESEJADO Q2 : PMIOPort  Port=2  Side=Right
  DESEJADO Q4 : PMIOPort  Port=3  Side=Right
  DESEJADO Q3 : PMIOPort  Port=4  Side=Right
  wires:
  [qd_dqd_d2qd] -> Bus Selector24/1
  Bus Selector24/3 -> Simulink-PS Converter6/3  "<d2q4d>"
  Bus Selector24/1 -> Simulink-PS Converter6/1  "<q4>"
  Bus Selector22/1 -> Simulink-PS Converter4/1  "<q1>"
  Bus Selector23/2 -> Simulink-PS Converter5/2  "<dq2d>"
  Bus Selector24/6 -> Simulink-PS Converter7/3  "<d2q3d>"
  [qd_dqd_d2qd] -> Bus Selector22/1
  Bus Selector23/3 -> Simulink-PS Converter5/3  "<d2q2d>"
  Bus Selector22/2 -> Simulink-PS Converter4/2  "<dq1d>"
  [qd_dqd_d2qd] -> Bus Selector23/1
  Bus Selector24/2 -> Simulink-PS Converter6/2  "<dq4d>"
  Bus Selector24/5 -> Simulink-PS Converter7/2  "<dq3d>"
  Bus Selector23/1 -> Simulink-PS Converter5/1  "<q2>"
  Bus Selector22/3 -> Simulink-PS Converter4/3  "<d2q1d>"
  Bus Selector24/4 -> Simulink-PS Converter7/1  "<q3>"
  connections:
  Simulink-PS Converter4/RConn1 -- DESEJADO Q1/RConn1
  Simulink-PS Converter5/RConn1 -- DESEJADO Q2/RConn1
  Simulink-PS Converter6/RConn1 -- DESEJADO Q4/RConn1
  Simulink-PS Converter7/RConn1 -- DESEJADO Q3/RConn1

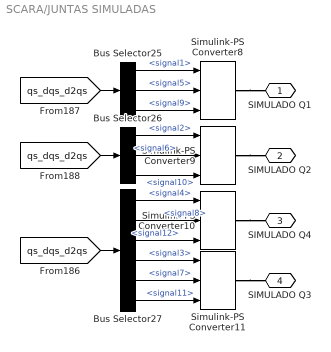
== system SCARA/JUNTAS SIMULADAS ==
  Bus Selector25 : BusSelector  OutputSignals=signal1,signal5,signal9
  Bus Selector26 : BusSelector  OutputSignals=signal2,signal6,signal10
  Bus Selector27 : BusSelector  OutputSignals=signal4,signal8,signal12,signal3,signal7,signal11
  Simulink-PS Converter{8..11} (4 alike) : nesl_utility/Simulink-PS Converter  PhysicalDomain=network_engine_domain  SubClassName=ps_input  LeftPortType=input  RightPortType=output  PseudoPeriodic=off  Frequencies=[]  NoiseDistribution=none  NoiseParameters=[]  Unit=1  AffineConversion=off  FilteringAndDerivatives=provide  SimscapeFilterOrder=1  InputFilterTimeConstant=0.001  UdotUserProvided=2
  SIMULADO Q1 : PMIOPort  Side=Right
  SIMULADO Q2 : PMIOPort  Port=2  Side=Right
  SIMULADO Q4 : PMIOPort  Port=3  Side=Right
  SIMULADO Q3 : PMIOPort  Port=4  Side=Right
  wires:
  Bus Selector26/2 -> Simulink-PS Converter9/2  "<signal6>"
  Bus Selector25/3 -> Simulink-PS Converter8/3  "<signal9>"
  [qs_dqs_d2qs] -> Bus Selector27/1
  Bus Selector26/3 -> Simulink-PS Converter9/3  "<signal10>"
  Bus Selector25/2 -> Simulink-PS Converter8/2  "<signal5>"
  Bus Selector27/4 -> Simulink-PS Converter11/1  "<signal3>"
  [qs_dqs_d2qs] -> Bus Selector26/1
  Bus Selector27/6 -> Simulink-PS Converter11/3  "<signal11>"
  Bus Selector27/2 -> Simulink-PS Converter10/2  "<signal8>"
  Bus Selector26/1 -> Simulink-PS Converter9/1  "<signal2>"
  Bus Selector27/1 -> Simulink-PS Converter10/1  "<signal4>"
  Bus Selector27/3 -> Simulink-PS Converter10/3  "<signal12>"
  Bus Selector27/5 -> Simulink-PS Converter11/2  "<signal7>"
  Bus Selector25/1 -> Simulink-PS Converter8/1  "<signal1>"
  [qs_dqs_d2qs] -> Bus Selector25/1
  connections:
  Simulink-PS Converter10/RConn1 -- SIMULADO Q4/RConn1
  Simulink-PS Converter8/RConn1 -- SIMULADO Q1/RConn1
  Simulink-PS Converter9/RConn1 -- SIMULADO Q2/RConn1
  Simulink-PS Converter11/RConn1 -- SIMULADO Q3/RConn1

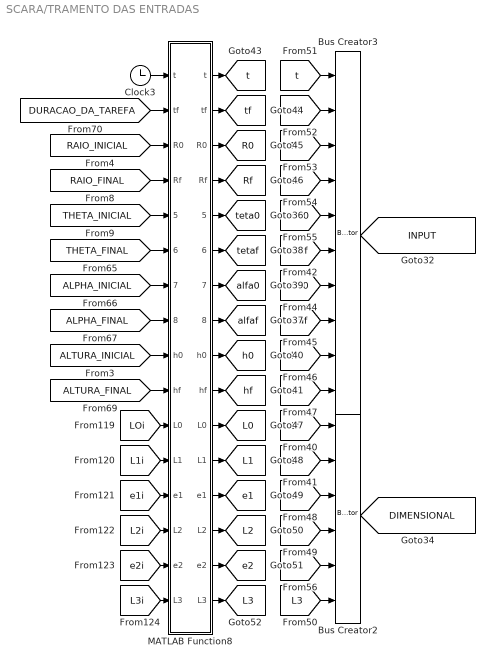
== system SCARA/TRAMENTO DAS ENTRADAS ==
  Bus Creator2 : BusCreator  Inputs=6
  Bus Creator3 : BusCreator  Inputs=10
  Clock3 : Clock
  MATLAB Function8 : MATLAB Function  TreatAsAtomicUnit=on
  tag scope: DIMENSIONAL=global, INPUT=global, L0=global, L1=global, L2=global, L3=global, R0=global, Rf=global, alfa0=global, alfaf=global, e1=global, e2=global, h0=global, hf=global, t=global, teta0=global, tetaf=global, tf=global
  wires:
  MATLAB Function8/15(e2) -> [e2]
  [LOi] -> MATLAB Function8/11("L0 ")
  MATLAB Function8/5(teta0) -> [teta0]
  [DURACAO_DA_TAREFA] -> MATLAB Function8/2("tf ")
  [Rf] -> Bus Creator3/4
  [L2i] -> MATLAB Function8/14("L2 ")
  [tetaf] -> Bus Creator3/6
  [ALPHA_INICIAL] -> MATLAB Function8/7("alfa0 ")
  [ALTURA_INICIAL] -> MATLAB Function8/9("h0 ")
  [R0] -> Bus Creator3/3
  [e2i] -> MATLAB Function8/15("e2 ")
  [L1] -> Bus Creator2/2
  MATLAB Function8/8(alfaf) -> [alfaf]
  [L0] -> Bus Creator2/1
  MATLAB Function8/2(tf) -> [tf]
  Bus Creator2/1 -> [DIMENSIONAL]
  [e2] -> Bus Creator2/5
  [alfaf] -> Bus Creator3/8
  MATLAB Function8/4(Rf) -> [Rf]
  MATLAB Function8/1(t) -> [t]
  [L3] -> Bus Creator2/6
  [t] -> Bus Creator3/1
  [ALPHA_FINAL] -> MATLAB Function8/8("alfaf ")
  [THETA_FINAL] -> MATLAB Function8/6("tetaf ")
  [L1i] -> MATLAB Function8/12("L1 ")
  MATLAB Function8/7(alfa0) -> [alfa0]
  MATLAB Function8/9(h0) -> [h0]
  [hf] -> Bus Creator3/10
  Bus Creator3/1 -> [INPUT]
  [ALTURA_FINAL] -> MATLAB Function8/10("hf ")
  [e1] -> Bus Creator2/3
  [h0] -> Bus Creator3/9
  MATLAB Function8/14(L2) -> [L2]
  MATLAB Function8/6(tetaf) -> [tetaf]
  MATLAB Function8/12(L1) -> [L1]
  MATLAB Function8/13(e1) -> [e1]
  MATLAB Function8/3(R0) -> [R0]
  MATLAB Function8/11(L0) -> [L0]
  [RAIO_FINAL] -> MATLAB Function8/4("Rf ")
  [L2] -> Bus Creator2/4
  Clock3/1 -> MATLAB Function8/1("t ")
  MATLAB Function8/16(L3) -> [L3]
  [THETA_INICIAL] -> MATLAB Function8/5("teta0 ")
  [teta0] -> Bus Creator3/5
  [e1i] -> MATLAB Function8/13("e1 ")
  [alfa0] -> Bus Creator3/7
  MATLAB Function8/10(hf) -> [hf]
  [L3i] -> MATLAB Function8/16("L3 ")
  [tf] -> Bus Creator3/2
  [RAIO_INICIAL] -> MATLAB Function8/3("R0 ")

== matlab function SCARA/MATLAB Function1 ==
  data: horario input; x output; q1 input; y output; q2 input; q3 input; q4 input; z output; L0 input; L1 input; e1 input; L2 input
function [x,y,z] = teste_da_cinematica_inversa(horario,q1,q2,q3,q4,L0,L1,e1,L2)

% if horario ==0
    x= L1*cos(q1)+L2*cos(q1+q2)
    y= L1*sin(q1)+L2*sin(q1+q2)
    z= L0+e1+q3
% else
%     x= L1*cos(q1)+L2*cos(q1-q2)
%     y= L1*sin(q1)+L2*sin(q1-q2)
%     z= L0+e1+q3
% end
end

== matlab function SCARA/VALORES ==
  data: LOi output; L1i output; e1i output; L2i output; e2i output; L3i output; c1 output; c2 output; c3 output; c4 output; g output; m1 output; xG1 output; yG1 output; zG1 output; Ixx1 output; Ixy1 output; Ixz1 output; Iyy1 output; Iyz1 output; Izz1 output; m2 output; xG2 output; yG2 output; zG2 output; Ixx2 output; Ixy2 output; Ixz2 output; Iyy2 output; Iyz2 output; Izz2 output; m3 output; xG3 output; yG3 output; zG3 output; Ixx3 output; Ixy3 output; Ixz3 output; Iyy3 output; Iyz3 output; Izz3 output
function [LOi, L1i, e1i, L2i, e2i, L3i, c1, c2, c3, c4, g, m1, xG1, yG1, zG1, Ixx1 ,Ixy1, Ixz1, Iyy1, Iyz1, Izz1, m2, xG2, yG2, zG2, Ixx2, Ixy2, Ixz2, Iyy2, Iyz2, Izz2, m3, xG3, yG3, zG3, Ixx3, Ixy3, Ixz3, Iyy3, Iyz3, Izz3 ]   = VALORES

%%
LOi = 0.5;
L1i = 0.5;
e1i = 0.1;  
L2i = 0.5;
e2i = 0.1;
L3i = 0.5;
c1 = 0.1; c2 = 0.1; c3 = 0.1; c4 = 0.1;
g = 9.80665;


%% CONSTANTES PARA O ELO 1
% ELO 01 SCARA
% 
% Massa = 390.51360 quilogramas
% 
% Centro de massa: ( metros )
% 	X = -0.03700
% 	Y = 0.00000
% 	Z = 0.08330
% 
% Momentos de inércia: ( quilogramas * metros quadrados )
% Tomados no sistema de coordenadas de saída.
% 	Ixx = 9.96587	Ixy = 0.00000	Ixz = -5.90046
% 	Iyx = 0.00000	Iyy = 29.92463	Iyz = 0.00000
% 	Izx = -5.90046	Izy = 0.00000	Izz = 27.17201

m1 = 390.51360;
xG1 = -0.03700;
yG1 = 0.00;
zG1 = 0.08330;
Ixx1 = 9.96587 ; Ixy1 = 0.00 ; Ixz1 = -5.90046 ; Iyy1 = 29.92463 ; Iyz1 = 0.00 ; Izz1 = 27.17201;


%% CONSTANTES PARA O ELO 2

% % Propriedades de massa de ELO 02 SCARA izz
% %      Configuração: Valor predeterminado
% %      Sistema de coordenadas: Sistema de coordenadas1
% % 
% % Densidade = 7850.0000 quilogramas por metro cúbico
% % 
% % Massa = 210.9470 quilogramas
% % 
% % Volume = 0.0269 metros cúbicos
% % 
% % Área de superfície = 0.8731 metros quadrados
% % 
% % Centro de massa: ( metros )
% % 	X = -0.2116
% % 	Y = 0.0000
% % 	Z = 0.0000
% % 
% % Eixos principais de inércia e momentos de inércia principais: ( quilogramas * metros quadrados )
% % Tomado no centro da massa.
% % 	 Ix = ( 1.0000,  0.0000,  0.0000)   	Px = 3.1012
% % 	 Iy = ( 0.0000,  1.0000,  0.0000)   	Py = 11.5266
% % 	 Iz = ( 0.0000,  0.0000,  1.0000)   	Pz = 14.2763
% % 
% % Momentos de inércia: ( quilogramas * metros quadrados )
% % Obtido no centro de massa e alinhado com o sistema de coordenadas de saída.
% % 	Lxx = 3.1012	Lxy = 0.0000	Lxz = 0.0000
% % 	Lyx = 0.0000	Lyy = 11.5266	Lyz = 0.0000
% % 	Lzx = 0.0000	Lzy = 0.0000	Lzz = 14.2763
% % 
% % Momentos de inércia: ( quilogramas * metros quadrados )
% % Tomados no sistema de coordenadas de saída.
% % 	Ixx = 3.1012	Ixy = 0.0000	Ixz = 0.0000
% % 	Iyx = 0.0000	Iyy = 20.9752	Iyz = 0.0000
% % 	Izx = 0.0000	Izy = 0.0000	Izz = 23.7249

m2 = 210.9470;
xG2 = -0.2116;
yG2 = 0.00;
zG2 = 0.00;
Ixx2 = 3.1012 ; Ixy2 = 0.00 ; Ixz2 = 0.0 ; Iyy2 = 20.9752 ; Iyz2 = 0.00 ; Izz2 = 23.7249;

%% CONSTANTES PARA O ELO 3
% Propriedades de massa de ELO 03 SCARA_Valor predeterminado_sldprt
%      Configuração: Valor predeterminado
%      Sistema de coordenadas: Sistema de coordenadas1
% 
% Densidade = 7850.0000 quilogramas por metro cúbico
% 
% Massa = 98.0685 quilogramas
% 
% Volume = 0.0125 metros cúbicos
% 
% Área de superfície = 0.5204 metros quadrados
% 
% Centro da massa (substituído pelo usuário): ( metros )
% 	X = 0.0000
% 	Y = 0.0000
% 	Z = 0.1965
% 
% Eixos principais de inércia e momentos de inércia principais: ( quilogramas * metros quadrados )
% Tomado no centro da massa.
% 	 Ix = ( 0.0000,  0.0000,  1.0000)   	Px = 0.8586
% 	 Iy = ( 1.0000,  0.0000,  0.0000)   	Py = 7.8563
% 	 Iz = ( 0.0000,  1.0000,  0.0000)   	Pz = 8.5694
% 
% Momentos de inércia: ( quilogramas * metros quadrados )
% Obtido no centro de massa e alinhado com o sistema de coordenadas de saída.
% 	Lxx = 7.8563	Lxy = 0.0000	Lxz = 0.0000
% 	Lyx = 0.0000	Lyy = 8.5694	Lyz = 0.0000
% 	Lzx = 0.0000	Lzy = 0.0000	Lzz = 0.8586
% 
% Momentos de inércia: ( quilogramas * metros quadrados )
% Tomados no sistema de coordenadas de saída.


m3 = 98.0685;
xG3 = 0.0000;
yG3 = 0.0000;
zG3 = 0.1965;
Ixx3 = 11.6437 ; Ixy3 =0 ; Ixz3 =0 ; Iyy3 = 12.3568 ; Iyz3 =0 ; Izz3 = 0.8586;

== matlab function SCARA/D ==
  data: c1 input; D output; c2 input; c3 input; c4 input; dq1 input; dq2 input; dq3 input; dq4 input
function D = D(c1,c2,c3,c4,dq1,dq2,dq3,dq4)
%#codegen

%    This function was generated by the Symbolic Math Toolbox version 8.6.
%    30-Apr-2021 16:43:50

D = [c1.*dq1;c2.*dq2;c3.*dq3.^2.*(3.0./2.0);c4.*dq4];

== matlab function SCARA/G ==
  data: g input; G output; m3 input
function G = G(g,m3)
%#codegen

%    This function was generated by the Symbolic Math Toolbox version 8.6.
%    30-Apr-2021 16:43:50

G = [0.0;0.0;g.*m3;0.0];

== matlab function SCARA/H ==
  data: L1 input; H output; L2 input; dq1 input; dq2 input; dq4 input; m2 input; m3 input; q2 input; q4 input; xG2 input; xG3 input; yG2 input; yG3 input
function H = H(L1,L2,dq1,dq2,dq4,m2,m3,q2,q4,xG2,xG3,yG2,yG3)


t2 = cos(q2);
t3 = cos(q4);
t4 = sin(q2);
t5 = sin(q4);
t6 = q2+q4;
t7 = dq1.^2;
t8 = dq2.^2;
t9 = dq4.^2;
t10 = cos(t6);
t11 = sin(t6);
t12 = L2.*m3.*t3.*t9.*yG3;
t13 = L2.*dq1.*dq4.*m3.*t3.*yG3.*2.0;
t14 = L2.*dq2.*dq4.*m3.*t3.*yG3.*2.0;
t15 = L2.*m3.*t5.*t9.*xG3;
t16 = L2.*dq1.*dq4.*m3.*t5.*xG3.*2.0;
t17 = L2.*dq2.*dq4.*m3.*t5.*xG3.*2.0;
t18 = -t13;
t19 = -t14;
t20 = -t16;
t21 = -t17;
t22 = -t12;
t23 = -t15;
H = [t18+t19+t20+t21+t22+t23-L1.*L2.*m2.*t4.*t8-L1.*L2.*m3.*t4.*t8-L1.*m2.*t4.*t8.*xG2-L1.*m3.*t8.*t11.*xG3-L1.*m3.*t9.*t11.*xG3-L1.*m2.*t2.*t8.*yG2-L1.*m3.*t8.*t10.*yG3-L1.*m3.*t9.*t10.*yG3-L1.*L2.*dq1.*dq2.*m2.*t4.*2.0-L1.*L2.*dq1.*dq2.*m3.*t4.*2.0-L1.*dq1.*dq2.*m2.*t4.*xG2.*2.0-L1.*dq1.*dq2.*m3.*t11.*xG3.*2.0-L1.*dq1.*dq4.*m3.*t11.*xG3.*2.0-L1.*dq2.*dq4.*m3.*t11.*xG3.*2.0-L1.*dq1.*dq2.*m2.*t2.*yG2.*2.0-L1.*dq1.*dq2.*m3.*t10.*yG3.*2.0-L1.*dq1.*dq4.*m3.*t10.*yG3.*2.0-L1.*dq2.*dq4.*m3.*t10.*yG3.*2.0;t18+t19+t20+t21+t22+t23+L1.*L2.*m2.*t4.*t7+L1.*L2.*m3.*t4.*t7+L1.*m2.*t4.*t7.*xG2+L1.*m3.*t7.*t11.*xG3+L1.*m2.*t2.*t7.*yG2+L1.*m3.*t7.*t10.*yG3;0.0;m3.*(L2.*t5.*t7.*xG3+L2.*t5.*t8.*xG3+L1.*t7.*t11.*xG3+L2.*t3.*t7.*yG3+L2.*t3.*t8.*yG3+L1.*t7.*t10.*yG3+L2.*dq1.*dq2.*t5.*xG3.*2.0+L2.*dq1.*dq2.*t3.*yG3.*2.0)];
